simulink model "a8_real_control_smc"  (R2023b)
settings: Solver=FixedStepAuto  StartTime=0.0  StopTime=inf  RelTol=1e-3
undefined symbols (not defined in the file): dev, Main, pid_y_i, pwm_output0
libraries: simulink x15, slpidlib x6, px4Sensorslib x5, px4lib x1, px4uORBlib x1
(part 1 of 2)
settings Model: SimulationMode=external  ExtModeTrigDuration=10  Creator=UAV2  LastModifiedBy=UAV2
settings SolverCC: AlgebraicLoopSolver=TrustRegion  PositivePriorityOrder=on  MaxZcPerStep=1
settings OptimizationCC: EnhancedBackFolding=on  PassReuseOutputArgsAs=Individual arguments  ZeroExternalMemoryAtStartup=off  ZeroInternalMemoryAtStartup=off  MaxStackSize=64  OptimizeBlockOrder=speed  DifferentSizesBufferReuse=on  OptimizationCustomize=off  EfficientTunableParamExpr=on
settings DebuggingCC: ParameterTunabilityLossMsg=error  UnconnectedInputMsg=warning  UnconnectedOutputMsg=warning  UnconnectedLineMsg=warning  SymbolicDimsDataTypeCodeGenerationDiagnostic=none
settings HardwareCC: ProdBitPerPointer=32  ProdBitPerSizeT=32  ProdBitPerPtrDiffT=32  ProdLargestAtomicInteger=Long  ProdLargestAtomicFloat=Double  ProdWordSize=32  ProdLongLongMode=on  ProdHWDeviceType=ARM Compatible->ARM Cortex
settings ModelReferenceCC: EnableRefExpFcnMdlSchedulingChecks=on
settings SFSimCC: SimGenImportedTypeDefs=on  MATLABDynamicMemAlloc=off  SimTargetLang=C++
settings RTWCC: Description=Embedded Coder  SystemTargetFile=ert.tlc  HardwareBoard=PX4 Pixhawk 4  TemplateMakefile=ert_default_tmf  Toolchain=GNU Tools for PX4 Autopilots  IncludeHyperlinkInReport=on  TargetLang=C++  DLArmComputeVersion=19.05
settings CodeAppCC: ForceParamTrailComments=on  IgnoreCustomStorageClasses=off  OperatorAnnotations=on  SimulinkDataObjDesc=on  SFDataObjDesc=on  InsertBlockDesc=on
settings ERTTargetCC: ExtMode=on  ExtModeTransport=3  ExtModeStaticAlloc=on  ExtModeStaticAllocSize=1024  ExtModeMexFile=ext_xcp  ExtModeMexArgs=1 COM3 3000000  ExtModeIntrfLevel=Level2 - Open

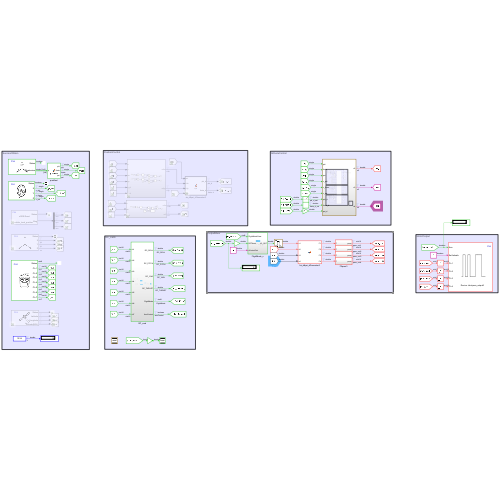
[thumbnail: Simulink's stored preview of the top-level diagram]
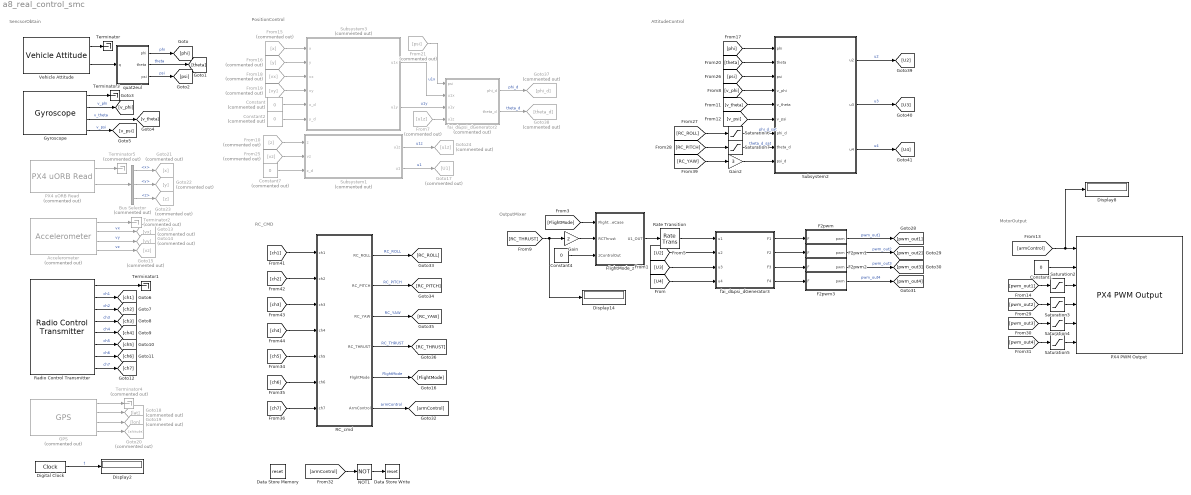
== system a8_real_control_smc ==
  note: RC_CMD
  note: PositionControl
  note: MotorOutput
  note: SencsorObtain
  note: AttitudeControl
  note: OutputMixer
  Accelerometer : px4Sensorslib/Accelerometer  Commented=on  uorbTimeStamp=off  BlockingMode=off  BlockTimeout=1e-3  sampleTime=1/250
  Bus Selector : BusSelector  Commented=on  OutputSignals=x,y,z
  Constant : Constant  Commented=on  Value=0
  Constant1 : Constant  Value=0  OutDataTypeStr=boolean
  Constant2 : Constant  Commented=on  Value=0
  Constant4 : Constant  Value=0  OutDataTypeStr=double
  Constant7 : Constant  Commented=on  Value=0
  Data Store Memory : DataStoreMemory  DataStoreName=reset  WriteAfterWriteMsg=warning  ShowAdditionalParam=off  OutDataTypeStr=boolean
  Data Store Write : DataStoreWrite  DataStoreName=reset  IndexOptions=Index vector (dialog)  Indices=1  OutputSizes=1
  Digital Clock : DigitalClock  SampleTime=0.001
  Display14 : Display
  Display2 : Display
  Display8 : Display
  F2pwm : Subsystem
  F2pwm1 : Subsystem
  F2pwm2 : Subsystem
  F2pwm3 : Subsystem
  FlightMode_z : Subsystem
  From10 : From  Commented=on  GotoTag=z
  From15 : From  Commented=on  GotoTag=x
  From16 : From  Commented=on  GotoTag=y
  From18 : From  Commented=on  GotoTag=vx
  From19 : From  Commented=on  GotoTag=vy
  From21 : From  Commented=on  GotoTag=psi
  From25 : From  Commented=on  GotoTag=vz
  From7 : From  Commented=on  GotoTag=u1z
  GPS : px4Sensorslib/GPS  Commented=on  lat=on  lon=on  alt=on  velocity=off  course=off  gpsfix=off  numsat=off  timestamp_utc=off  BlockingMode=off  BlockTimeout=1e-3  dop=off  vel_ned=off  alt_ellipsoid=off  jamm_ind=off  timestamp=off  sampleTime=1/250
  Gain : Gain  Gain=2
  Gain2 : Gain  Gain=3
  Goto13 : Goto  Commented=on  GotoTag=vx
  Goto14 : Goto  Commented=on  GotoTag=vy
  Goto15 : Goto  Commented=on  GotoTag=vz
  Goto17 : Goto  Commented=on  GotoTag=U1
  Goto18 : Goto  Commented=on  GotoTag=lat
  Goto19 : Goto  Commented=on  GotoTag=lon
  Goto20 : Goto  Commented=on  GotoTag=altitude
  Goto21 : Goto  Commented=on  GotoTag=x
  Goto22 : Goto  Commented=on  GotoTag=y
  Goto23 : Goto  Commented=on  GotoTag=z
  Goto24 : Goto  Commented=on  GotoTag=u1z
  Goto37 : Goto  Commented=on  GotoTag=phi_d
  Goto38 : Goto  Commented=on  GotoTag=theta_d
  Gyroscope : px4Sensorslib/Gyroscope  uorbTimeStamp=off  BlockingMode=off  BlockTimeout=1e-3  sampleTime=1/250
  NOT1 : Logic  Operator=NOT  IconShape=distinctive  AllPortsSameDT=off  OutDataTypeStr=boolean
  PX4 PWM Output : px4lib/PX4 PWM Output  pwmDevice=Main (/dev/pwm_output0)  pwmChannel1_=on  pwmChannel2_=on  pwmChannel3_=on  pwmChannel4_=on  pwmChannel5_=off  pwmChannel6_=off  pwmChannel7_=off  pwmChannel8_=off  forceTerminateFailsafe=off  outputErrorStatus=off
  PX4 uORB Read : px4uORBlib/PX4 uORB Read  Commented=on  uORBTopic=vehicle_local_position  selectInstance=actuator_armed  SampleTime=1/250  BlockingMode=off  BlockTimeout=1e-3
  RC_cmd : Subsystem  Tag=attitudeControl
  Radio Control Transmitter : px4Sensorslib/Radio Control Transmitter  channel1=on  channel2=on  channel3=on  channel4=on  channel5=on  channel6=on  channel7=on  channel8=off  channel_count=off  rssi=off  rc_input_source=off  timestamp_last_signal=off  time_stamp=off  sampleTime=1/250  BlockingMode=off  BlockTimeout=5
  Rate Transition : RateTransition
  Saturation{2..5} (4 alike) : Saturate  UpperLimit=2000  LowerLimit=1050
  Saturation6 : Saturate
  Saturation7 : Saturate
  Subsystem1 : Subsystem  Commented=on
  Subsystem2 : Subsystem
  Subsystem3 : Subsystem  Commented=on
  Terminator : Terminator
  Terminator1 : Terminator
  Terminator2 : Terminator  Commented=on
  Terminator3 : Terminator
  Terminator4 : Terminator  Commented=on
  Terminator5 : Terminator  Commented=on
  Vehicle Attitude : px4Sensorslib/Vehicle Attitude  rollRate=off  pitchRate=off  yawRate=off  quaternion=on  uorbTimeStamp=off  BlockingMode=off  BlockTimeout=0.001  sampleTime=1/250
  fai_d&psi_dGenerator2 : MATLAB Function  Commented=on  TreatAsAtomicUnit=on
  fai_d&psi_dGenerator3 : MATLAB Function  TreatAsAtomicUnit=on
  quat2eul : MATLAB Function  TreatAsAtomicUnit=on
  wires:
  Accelerometer/3 -> Goto14/1  "vy"
  [armControl] -> NOT1/1
  From19/1 -> Subsystem3/4(vy)
  Constant1/1 -> PX4 PWM Output/2
  [ch3] -> RC_cmd/3(ch3)
  Gyroscope/3 -> [v_theta]  "v_theta"
  [ch2] -> RC_cmd/2(ch2)
  quat2eul/2(theta) -> [theta]  "theta"
  [pwm_out3] -> Saturation4/1
  Constant2/1 -> Subsystem3/6(y_d)
  Gain/1 -> FlightMode_z/2(RCThrust)
  Constant/1 -> Subsystem3/5(x_d)
  fai_d&psi_dGenerator3/3(F3) -> F2pwm2/1(F)
  [ch6] -> RC_cmd/6(ch6)
  Bus Selector/3 -> Goto23/1  "<z>"
  [ch4] -> RC_cmd/4(ch4)
  FlightMode_z/1(U1_OUT) -> Rate Transition/1
  RC_cmd/5(FlightMode) -> [FlightMode]  "FlightMode"
  fai_d&psi_dGenerator2/2(theta_d) -> Goto38/1  "theta_d"
  Accelerometer/1 -> Terminator2/1
  Constant4/1 -> FlightMode_z/3(zControlOut)
  RC_cmd/6(ArmControl) -> [armControl]  "armControl"
  From16/1 -> Subsystem3/2(y)
  RC_cmd/1(RC_ROLL) -> [RC_ROLL]  "RC_ROLL"
  [RC_THRUST] -> Display14/1, Gain/1
  quat2eul/1(phi) -> [phi]  "phi"
  NOT1/1 -> Data Store Write/1
  RC_cmd/4(RC_THRUST) -> [RC_THRUST]  "RC_THRUST"
  Vehicle Attitude/2 -> quat2eul/1(q)
  RC_cmd/2(RC_PITCH) -> [RC_PITCH]  "RC_PITCH"
  RC_cmd/3(RC_YAW) -> [RC_YAW]  "RC_YAW"
  [ch5] -> RC_cmd/5(ch5)
  F2pwm/1(pwm) -> [pwm_out1]  "pwm_out1"
  [ch7] -> RC_cmd/7(ch7)
  [pwm_out1] -> Saturation2/1
  fai_d&psi_dGenerator3/2(F2) -> F2pwm1/1(F)
  [ch1] -> RC_cmd/1(ch1)
  F2pwm1/1(pwm) -> [pwm_out2]  "pwm_out2"
  [pwm_out2] -> Saturation3/1
  Radio Control Transmitter/2 -> [ch1]  "ch1"
  fai_d&psi_dGenerator3/4(F4) -> F2pwm3/1(F)
  Accelerometer/2 -> Goto13/1  "vx"
  fai_d&psi_dGenerator3/1(F1) -> F2pwm/1(F)
  [pwm_out4] -> Saturation5/1
  Accelerometer/4 -> Goto15/1  "vz"
  Subsystem3/1(u1x) -> fai_d&psi_dGenerator2/2(u1x)  "u1x"
  Subsystem3/2(u1y) -> fai_d&psi_dGenerator2/3(u1y)  "u1y"
  From18/1 -> Subsystem3/3(vx)
  From21/1 -> fai_d&psi_dGenerator2/1(psi)
  Bus Selector/2 -> Goto22/1  "<y>"
  Radio Control Transmitter/5 -> [ch4]  "ch4"
  Radio Control Transmitter/6 -> [ch5]  "ch5"
  Radio Control Transmitter/8 -> [ch7]  "ch7"
  Gyroscope/1 -> Terminator3/1
  Radio Control Transmitter/3 -> [ch2]  "ch2"
  PX4 uORB Read/2 -> Bus Selector/1
  Radio Control Transmitter/7 -> [ch6]  "ch6"
  GPS/4 -> Goto20/1
  Bus Selector/1 -> Goto21/1  "<x>"
  GPS/1 -> Terminator4/1
  From15/1 -> Subsystem3/1(x)
  quat2eul/3(psi) -> [psi]  "psi"
  Vehicle Attitude/1 -> Terminator/1
  Gyroscope/4 -> [v_psi]  "v_psi"
  F2pwm3/1(pwm) -> [pwm_out4]  "pwm_out4"
  [armControl] -> Display8/1, PX4 PWM Output/1
  Radio Control Transmitter/4 -> [ch3]  "ch3"
  fai_d&psi_dGenerator2/1(phi_d) -> Goto37/1  "phi_d"
  Digital Clock/1 -> Display2/1  "t"
  GPS/2 -> Goto18/1
  Radio Control Transmitter/1 -> Terminator1/1
  PX4 uORB Read/1 -> Terminator5/1
  Gyroscope/2 -> [v_phi]  "v_phi"
  GPS/3 -> Goto19/1
  F2pwm2/1(pwm) -> [pwm_out3]  "pwm_out3"
  [FlightMode] -> FlightMode_z/1(FlightModeCase)
  Saturation2/1 -> PX4 PWM Output/3
  Saturation3/1 -> PX4 PWM Output/4
  Saturation4/1 -> PX4 PWM Output/5
  Saturation5/1 -> PX4 PWM Output/6
  Rate Transition/1 -> fai_d&psi_dGenerator3/1(u1)
  [U2] -> fai_d&psi_dGenerator3/2(u2)
  Subsystem1/2(u1) -> Goto17/1  "u1"
  From10/1 -> Subsystem1/1(z)
  From25/1 -> Subsystem1/2(vz)
  Constant7/1 -> Subsystem1/3(z_d)
  Subsystem1/1(u1z) -> Goto24/1  "u1z"
  From7/1 -> fai_d&psi_dGenerator2/4(u1z)
  [RC_PITCH] -> Saturation7/1
  [RC_ROLL] -> Saturation6/1
  [RC_YAW] -> Gain2/1
  Gain2/1 -> Subsystem2/9(psi_d)
  Saturation6/1 -> Subsystem2/7(phi_d)  "phi_d_sat"
  Saturation7/1 -> Subsystem2/8(theta_d)  "theta_d_sat"
  [phi] -> Subsystem2/1(phi)
  [theta] -> Subsystem2/2(theta)
  [psi] -> Subsystem2/3(psi)
  [v_phi] -> Subsystem2/4(v_phi)
  [v_theta] -> Subsystem2/5(v_theta)
  [v_psi] -> Subsystem2/6(v_psi)
  Subsystem2/1(u2) -> [U2]  "u2"
  Subsystem2/2(u3) -> [U3]  "u3"
  Subsystem2/3(u4) -> [U4]  "u4"
  [U3] -> fai_d&psi_dGenerator3/3(u3)
  [U4] -> fai_d&psi_dGenerator3/4(u4)

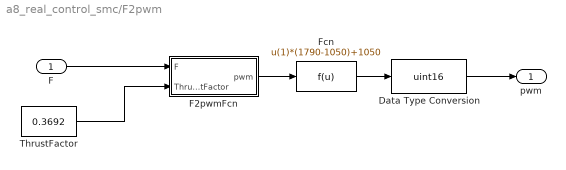
== system a8_real_control_smc/F2pwm ==
  F : Inport
  Data Type Conversion : DataTypeConversion  OutDataTypeStr=uint16  SaturateOnIntegerOverflow=off  RndMeth=Floor
  F2pwmFcn : Subsystem
  Fcn : Fcn  Expr=u(1)*(1790-1050)+1050
  ThrustFactor : Constant  Value=0.3692
  pwm : Outport  OutDataTypeStr=uint16  VectorParamsAs1DForOutWhenUnconnected=off
  wires:
  F/1 -> F2pwmFcn/1(F)
  ThrustFactor/1 -> F2pwmFcn/2(ThrustFactor)
  F2pwmFcn/1(pwm) -> Fcn/1
  Fcn/1 -> Data Type Conversion/1
  Data Type Conversion/1 -> pwm/1

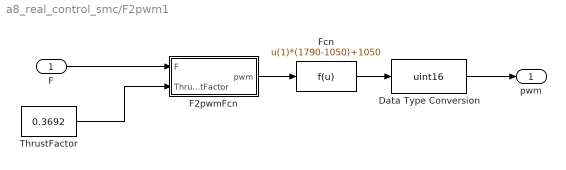
== system a8_real_control_smc/F2pwm1 ==
  F : Inport
  Data Type Conversion : DataTypeConversion  OutDataTypeStr=uint16  SaturateOnIntegerOverflow=off  RndMeth=Floor
  F2pwmFcn : Subsystem
  Fcn : Fcn  Expr=u(1)*(1790-1050)+1050
  ThrustFactor : Constant  Value=0.3692
  pwm : Outport  OutDataTypeStr=uint16  VectorParamsAs1DForOutWhenUnconnected=off
  wires:
  Data Type Conversion/1 -> pwm/1
  Fcn/1 -> Data Type Conversion/1
  F2pwmFcn/1(pwm) -> Fcn/1
  ThrustFactor/1 -> F2pwmFcn/2(ThrustFactor)
  F/1 -> F2pwmFcn/1(F)

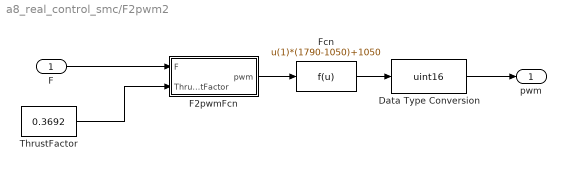
== system a8_real_control_smc/F2pwm2 ==
  F : Inport
  Data Type Conversion : DataTypeConversion  OutDataTypeStr=uint16  SaturateOnIntegerOverflow=off  RndMeth=Floor
  F2pwmFcn : Subsystem
  Fcn : Fcn  Expr=u(1)*(1790-1050)+1050
  ThrustFactor : Constant  Value=0.3692
  pwm : Outport  OutDataTypeStr=uint16  VectorParamsAs1DForOutWhenUnconnected=off
  wires:
  F/1 -> F2pwmFcn/1(F)
  ThrustFactor/1 -> F2pwmFcn/2(ThrustFactor)
  F2pwmFcn/1(pwm) -> Fcn/1
  Fcn/1 -> Data Type Conversion/1
  Data Type Conversion/1 -> pwm/1

== system a8_real_control_smc/F2pwm3 ==
  F : Inport
  Data Type Conversion : DataTypeConversion  OutDataTypeStr=uint16  SaturateOnIntegerOverflow=off  RndMeth=Floor
  F2pwmFcn : Subsystem
  Fcn : Fcn  Expr=u(1)*(1790-1050)+1050
  ThrustFactor : Constant  Value=0.3692
  pwm : Outport  OutDataTypeStr=uint16  VectorParamsAs1DForOutWhenUnconnected=off
  wires:
  Data Type Conversion/1 -> pwm/1
  Fcn/1 -> Data Type Conversion/1
  F2pwmFcn/1(pwm) -> Fcn/1
  ThrustFactor/1 -> F2pwmFcn/2(ThrustFactor)
  F/1 -> F2pwmFcn/1(F)

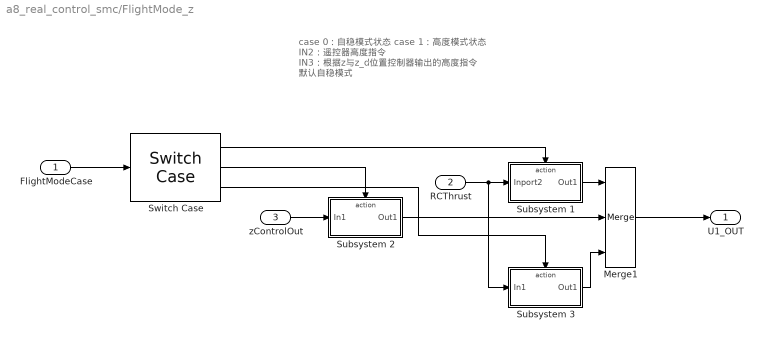
== system a8_real_control_smc/FlightMode_z ==
  note: case 0：自稳模式状态
      | case 1：高度模式状态
      | IN2：遥控器高度指令
      | IN3：根据z与z_d位置控制器输出的高度指令
      | 默认自稳模式
  FlightModeCase : Inport
  RCThrust : Inport  Port=2
  zControlOut : Inport  Port=3
  Merge1 : Merge  Inputs=3
  Subsystem 1 : Subsystem  TreatAsAtomicUnit=on
  Subsystem 2 : Subsystem  TreatAsAtomicUnit=on
  Subsystem 3 : Subsystem  TreatAsAtomicUnit=on
  Switch Case : SwitchCase  CaseConditions={0,1}
  U1_OUT : Outport  VectorParamsAs1DForOutWhenUnconnected=off
  wires:
  Switch Case/2 -> Subsystem 2/Action
  Subsystem 2/1(Out1) -> Merge1/2
  RCThrust/1 -> Subsystem 1/1(Inport2), Subsystem 3/1(In1)
  Switch Case/3 -> Subsystem 3/Action
  Subsystem 1/1(Out1) -> Merge1/1
  Switch Case/1 -> Subsystem 1/Action
  Subsystem 3/1(Out1) -> Merge1/3
  zControlOut/1 -> Subsystem 2/1(In1)
  FlightModeCase/1 -> Switch Case/1
  Merge1/1 -> U1_OUT/1

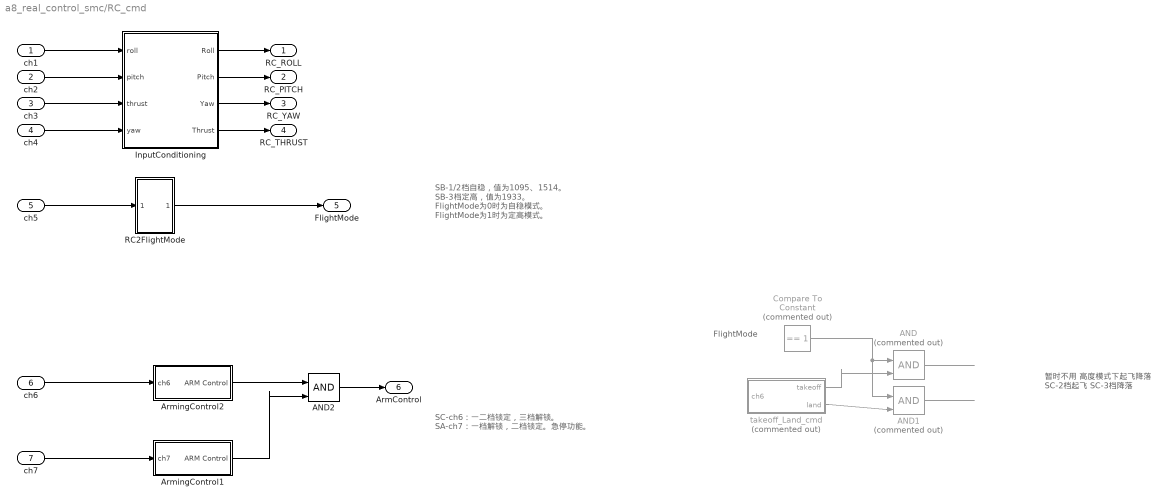
== system a8_real_control_smc/RC_cmd ==
  note: 暂时不用
      | 高度模式下起飞降落
      | SC-2档起飞
      | SC-3档降落
  note: SB-1/2档自稳，值为1095、1514。
      | SB-3档定高，值为1933。
      | FlightMode为0时为自稳模式。
      | FlightMode为1时为定高模式。
  note: FlightMode
  note: SC-ch6：一二档锁定，三档解锁。
      | SA-ch7：一档解锁，二档锁定。急停功能。
  ch1 : Inport  OutDataTypeStr=uint16
  ch2 : Inport  Port=2  OutDataTypeStr=uint16
  ch3 : Inport  Port=3  OutDataTypeStr=uint16
  ch4 : Inport  Port=4  OutDataTypeStr=uint16
  ch5 : Inport  Port=5  OutDataTypeStr=uint16
  ch6 : Inport  Port=6  OutDataTypeStr=uint16
  ch7 : Inport  Port=7  OutDataTypeStr=uint16
  AND : Logic  Commented=on  IconShape=distinctive  AllPortsSameDT=off  OutDataTypeStr=boolean
  AND1 : Logic  Commented=on  IconShape=distinctive  AllPortsSameDT=off  OutDataTypeStr=boolean
  AND2 : Logic  IconShape=distinctive  AllPortsSameDT=off  OutDataTypeStr=boolean
  ArmingControl1 : Subsystem
  ArmingControl2 : Subsystem
  Compare To Constant : simulink/Logic and Bit Operations/Compare To Constant  Commented=on  relop===  const=1  OutDataTypeStr=boolean
  InputConditioning : Subsystem
  RC2FlightMode : Subsystem
  takeoff_Land_cmd : Subsystem  Commented=on
  RC_ROLL : Outport
  RC_PITCH : Outport  Port=2
  RC_YAW : Outport  Port=3
  RC_THRUST : Outport  Port=4
  FlightMode : Outport  Port=5
  ArmControl : Outport  Port=6
  wires:
  ch7/1 -> ArmingControl1/1(ch7)
  ch4/1 -> InputConditioning/4(yaw)
  ch1/1 -> InputConditioning/1(roll)
  ch2/1 -> InputConditioning/2(pitch)
  ch3/1 -> InputConditioning/3(thrust)
  InputConditioning/1(Roll) -> RC_ROLL/1
  InputConditioning/2(Pitch) -> RC_PITCH/1
  InputConditioning/3(Yaw) -> RC_YAW/1
  InputConditioning/4(Thrust) -> RC_THRUST/1
  takeoff_Land_cmd/1(takeoff) -> AND/2
  AND/1 -> ?
  AND1/1 -> ?
  takeoff_Land_cmd/2(land) -> AND1/2
  ch5/1 -> RC2FlightMode/1(In1)
  RC2FlightMode/1(Out1) -> FlightMode/1
  Compare To Constant/1 -> AND1/1, AND/1
  ch6/1 -> ArmingControl2/1(ch6)
  ArmingControl2/1(ARM Control) -> AND2/1
  ArmingControl1/1(ARM Control) -> AND2/2
  AND2/1 -> ArmControl/1

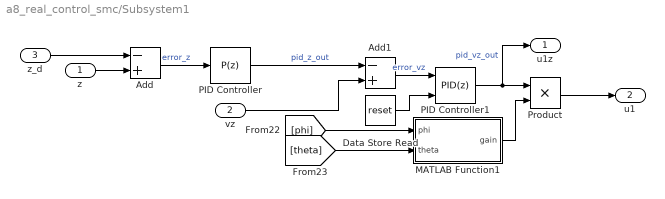
== system a8_real_control_smc/Subsystem1 ==
  z : Inport
  vz : Inport  Port=2
  z_d : Inport  Port=3
  Add : Sum  Inputs=-+
  Add1 : Sum  Inputs=-+
  Data Store Read : DataStoreRead  DataStoreName=reset  IndexOptions=Index vector (dialog)  Indices=1  OutputSizes=1
  MATLAB Function1 : MATLAB Function  TreatAsAtomicUnit=on
  PID Controller : slpidlib/PID Controller  Controller=P  Form=Parallel  TimeDomain=Discrete-time  UseExternalTs=off  SampleTime=-1  IntegratorMethod=Forward Euler  FilterMethod=Forward Euler  ControllerParametersSource=internal  P=1.5  I=1.33332542389365  UseKiTs=off  D=0.947452162670561  N=36.1071689779307  UseFilter=on  TunerSelectOption=Transfer Function Based (PID Tuner App)  InitialConditionSource=internal  InitialConditionForIntegrator=0  InitialConditionForFilter=0  DifferentiatorICPrevScaledInput=0  ExternalReset=none  TrackingMode=off  Kt=1  LimitOutput=on  SatLimitsSource=internal  UpperSaturationLimit=10  LowerSaturationLimit=-10  LinearizeAsGain=off  AntiWindupMode=none  Kb=1  LimitIntegrator=off  UpperIntegratorSaturationLimit=inf  LowerIntegratorSaturationLimit=-inf  POutMin=[]  POutMax=[]  IOutMin=[]  IOutMax=[]  DOutMin=[]  DOutMax=[]  NOutMin=[]  NOutMax=[]  SumOutMin=[]  SumOutMax=[]  SaturationOutMin=[]  SaturationOutMax=[]  PParamMin=[]  PParamMax=[]  IParamMin=[]  IParamMax=[]  DParamMin=[]  DParamMax=[]  NParamMin=[]  NParamMax=[]  KbParamMin=[]  KbParamMax=[]  KtParamMin=[]  KtParamMax=[]  KbOutMin=[]  KbOutMax=[]  KtOutMin=[]  KtOutMax=[]  IntegratorOutMin=[]  IntegratorOutMax=[]  FilterOutMin=[]  FilterOutMax=[]  SumI1OutMin=[]  SumI1OutMax=[]  SumI2OutMin=[]  SumI2OutMax=[]  SumI3OutMin=[]  SumI3OutMax=[]  SumI4OutMin=[]  SumI4OutMax=[]  SumDOutMin=[]  SumDOutMax=[]  DifferentiatorOutMin=[]  DifferentiatorOutMax=[]  FilterDiffOutCoefMin=[]  FilterDiffOutCoefMax=[]  ReciprocalOutMin=[]  ReciprocalOutMax=[]  SumDenOutMin=[]  SumDenOutMax=[]  SumNumOutMin=[]  SumNumOutMax=[]  DivideOutMin=[]  DivideOutMax=[]  UdiffTsProdOutMin=[]  UdiffTsProdOutMax=[]  NTsProdOutMin=[]  NTsProdOutMax=[]  UintegralTsProdOutMin=[]  UintegralTsProdOutMax=[]  UngainTsProdOutMin=[]  UngainTsProdOutMax=[]  ClampingZeroOutDataTypeStr=Inherit: Inherit via back propagation  ClampingZeroOutMin=[]  ClampingZeroOutMax=[]  FilterDenConstantOutDataTypeStr=Inherit: Inherit via back propagation  FilterDenConstantOutMin=[]  FilterDenConstantOutMax=[]  PCopyOutDataTypeStr=Inherit: Inherit via back propagation  PCopyOutMin=[]  PCopyOutMax=[]  NCopyOutDataTypeStr=Inherit: Inherit via back propagation  NCopyOutMin=[]  NCopyOutMax=[]  IntegratorContinuousStateAttributes=''  IntegratorStateMustResolveToSignalObject=off  IntegratorRTWStateStorageClass=Auto  FilterContinuousStateAttributes=''  FilterStateMustResolveToSignalObject=off  FilterRTWStateStorageClass=Auto  ParallelPVariant=InternalParameters  IdealPVariant=Disabled  IVariant=Disabled  DVariant=Disabled  IntegratorVariant=Disabled  SatVariant=Enabled  AWVariant=Disabled  PCopyVariant=Disabled  TRVariant=Disabled  FdbkBlocksVariant=Forward  IdealPFdbkVariant=Disabled  SatFdbkVariant=Disabled  DerivativeFilterVariant=Disabled  NVariant=Disabled  NCopyVariant=Disabled_SignalSpec  FilterICVariant=Disabled  IntegratorICVariant=Disabled  ExternalResetVariant=Disabled  TRSumVariant=Passthrough  SumFdbkVariant=Disabled  SumVariant=Passthrough_P  TsampFilterVariant=InternalTs  TsampNgainVariant=Passthrough  TsampIntegralVariant=Disabled_SignalSpec  ExternalSaturationOutDataTypeStr=Inherit: Same as second input
  PID Controller1 : slpidlib/PID Controller  Controller=PID  Form=Parallel  TimeDomain=Discrete-time  UseExternalTs=off  SampleTime=-1  IntegratorMethod=Forward Euler  FilterMethod=Forward Euler  ControllerParametersSource=internal  P=0.6  I=0.3  UseKiTs=off  D=0  N=10  UseFilter=on  TunerSelectOption=Transfer Function Based (PID Tuner App)  InitialConditionSource=internal  InitialConditionForIntegrator=0  InitialConditionForFilter=0  DifferentiatorICPrevScaledInput=0  ExternalReset=level  TrackingMode=off  Kt=1  LimitOutput=on  SatLimitsSource=internal  UpperSaturationLimit=1  LowerSaturationLimit=0  LinearizeAsGain=off  AntiWindupMode=none  Kb=1  LimitIntegrator=off  UpperIntegratorSaturationLimit=0.1  LowerIntegratorSaturationLimit=-0.1  POutMin=[]  POutMax=[]  IOutMin=[]  IOutMax=[]  DOutMin=[]  DOutMax=[]  NOutMin=[]  NOutMax=[]  SumOutMin=[]  SumOutMax=[]  SaturationOutMin=[]  SaturationOutMax=[]  PParamMin=[]  PParamMax=[]  IParamMin=[]  IParamMax=[]  DParamMin=[]  DParamMax=[]  NParamMin=[]  NParamMax=[]  KbParamMin=[]  KbParamMax=[]  KtParamMin=[]  KtParamMax=[]  KbOutMin=[]  KbOutMax=[]  KtOutMin=[]  KtOutMax=[]  IntegratorOutMin=[]  IntegratorOutMax=[]  FilterOutMin=[]  FilterOutMax=[]  SumI1OutMin=[]  SumI1OutMax=[]  SumI2OutMin=[]  SumI2OutMax=[]  SumI3OutMin=[]  SumI3OutMax=[]  SumI4OutMin=[]  SumI4OutMax=[]  SumDOutMin=[]  SumDOutMax=[]  DifferentiatorOutMin=[]  DifferentiatorOutMax=[]  FilterDiffOutCoefMin=[]  FilterDiffOutCoefMax=[]  ReciprocalOutMin=[]  ReciprocalOutMax=[]  SumDenOutMin=[]  SumDenOutMax=[]  SumNumOutMin=[]  SumNumOutMax=[]  DivideOutMin=[]  DivideOutMax=[]  UdiffTsProdOutMin=[]  UdiffTsProdOutMax=[]  NTsProdOutMin=[]  NTsProdOutMax=[]  UintegralTsProdOutMin=[]  UintegralTsProdOutMax=[]  UngainTsProdOutMin=[]  UngainTsProdOutMax=[]  ClampingZeroOutDataTypeStr=Inherit: Inherit via back propagation  ClampingZeroOutMin=[]  ClampingZeroOutMax=[]  FilterDenConstantOutDataTypeStr=Inherit: Inherit via back propagation  FilterDenConstantOutMin=[]  FilterDenConstantOutMax=[]  PCopyOutDataTypeStr=Inherit: Inherit via back propagation  PCopyOutMin=[]  PCopyOutMax=[]  NCopyOutDataTypeStr=Inherit: Inherit via back propagation  NCopyOutMin=[]  NCopyOutMax=[]  IntegratorContinuousStateAttributes=''  IntegratorStateMustResolveToSignalObject=off  IntegratorRTWStateStorageClass=Auto  FilterContinuousStateAttributes=''  FilterStateMustResolveToSignalObject=off  FilterRTWStateStorageClass=Auto  ParallelPVariant=InternalParameters  IdealPVariant=Disabled  IVariant=InternalParameters  DVariant=InternalParameters  IntegratorVariant=Discrete  SatVariant=Enabled  AWVariant=Passthrough  PCopyVariant=Disabled  TRVariant=Disabled  FdbkBlocksVariant=Forward  IdealPFdbkVariant=Disabled  SatFdbkVariant=Disabled  DerivativeFilterVariant=ForwardEulerFilter  NVariant=InternalParameters  NCopyVariant=Disabled  FilterICVariant=InternalICsFilter  IntegratorICVariant=InternalICs  ExternalResetVariant=ExternalReset  TRSumVariant=Passthrough  SumFdbkVariant=Disabled  SumVariant=Sum_PID  TsampFilterVariant=InternalTs  TsampNgainVariant=Passthrough  TsampIntegralVariant=Disabled_SignalSpec  ExternalSaturationOutDataTypeStr=Inherit: Same as second input
  Product : Product
  u1z : Outport
  u1 : Outport  Port=2
  wires:
  z/1 -> Add/2
  z_d/1 -> Add/1
  Data Store Read/1 -> PID Controller1/2
  Add1/1 -> PID Controller1/1  "error_vz"
  PID Controller/1 -> Add1/1  "pid_z_out"
  PID Controller1/1 -> Product/1, u1z/1  "pid_vz_out"
  vz/1 -> Add1/2
  MATLAB Function1/1(gain) -> Product/2
  [theta] -> MATLAB Function1/2(theta)
  Product/1 -> u1/1
  Add/1 -> PID Controller/1  "error_z"
  [phi] -> MATLAB Function1/1(phi)

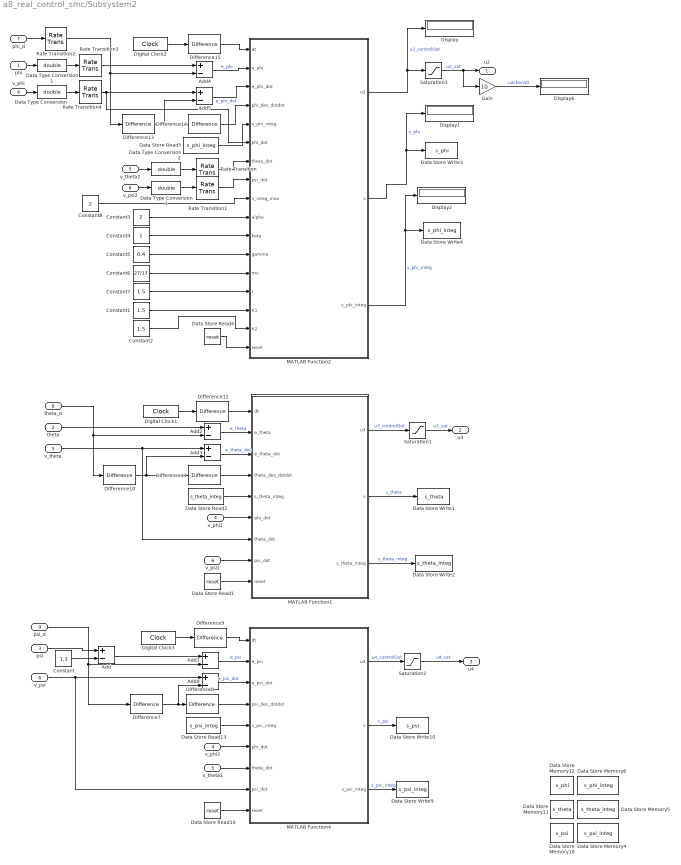
== system a8_real_control_smc/Subsystem2 ==
  phi : Inport
  theta : Inport  Port=2
  psi : Inport  Port=3
  v_phi : Inport  Port=4
  v_theta : Inport  Port=5
  v_psi : Inport  Port=6
  phi_d : Inport  Port=7
  theta_d : Inport  Port=8
  psi_d : Inport  Port=9
  Add{,1..5,9} (7 alike) : Sum  Inputs=+-
  Constant : Constant  Value=1.1
  Constant1 : Constant  Value=1.5
  Constant2 : Constant  Value=1.5
  Constant3 : Constant  Value=2
  Constant4 : Constant
  Constant5 : Constant  Value=0.4
  Constant6 : Constant  Value=27/17
  Constant7 : Constant  Value=1.5
  Constant8 : Constant  Value=2
  Data Store Memory10 : DataStoreMemory  DataStoreName=s_psi  WriteAfterWriteMsg=warning  ShowAdditionalParam=off  OutDataTypeStr=double
  Data Store Memory11 : DataStoreMemory  DataStoreName=s_theta  WriteAfterWriteMsg=warning  ShowAdditionalParam=off  OutDataTypeStr=double
  Data Store Memory12 : DataStoreMemory  DataStoreName=s_phi  WriteAfterWriteMsg=warning  ShowAdditionalParam=off  OutDataTypeStr=double
  Data Store Memory4 : DataStoreMemory  DataStoreName=s_psi_integ  WriteAfterWriteMsg=warning  ShowAdditionalParam=off  OutDataTypeStr=double
  Data Store Memory5 : DataStoreMemory  DataStoreName=s_theta_integ  WriteAfterWriteMsg=warning  ShowAdditionalParam=off  OutDataTypeStr=double
  Data Store Memory6 : DataStoreMemory  DataStoreName=s_phi_integ  WriteAfterWriteMsg=warning  ShowAdditionalParam=off  OutDataTypeStr=double
  Data Store Read1 : DataStoreRead  DataStoreName=reset  IndexOptions=Index vector (dialog)  Indices=1  OutputSizes=1
  Data Store Read10 : DataStoreRead  DataStoreName=reset  IndexOptions=Index vector (dialog)  Indices=1  OutputSizes=1
  Data Store Read13 : DataStoreRead  DataStoreName=s_psi_integ  IndexOptions=Index vector (dialog)  Indices=1  OutputSizes=1
  Data Store Read2 : DataStoreRead  DataStoreName=s_theta_integ  IndexOptions=Index vector (dialog)  Indices=1  OutputSizes=1
  Data Store Read4 : DataStoreRead  DataStoreName=reset  IndexOptions=Index vector (dialog)  Indices=1  OutputSizes=1
  Data Store Read5 : DataStoreRead  DataStoreName=s_phi_integ  IndexOptions=Index vector (dialog)  Indices=1  OutputSizes=1
  Data Store Write1 : DataStoreWrite  DataStoreName=s_theta  IndexOptions=Index vector (dialog)  Indices=1  OutputSizes=1
  Data Store Write10 : DataStoreWrite  DataStoreName=s_psi  IndexOptions=Index vector (dialog)  Indices=1  OutputSizes=1
  Data Store Write2 : DataStoreWrite  DataStoreName=s_theta_integ  IndexOptions=Index vector (dialog)  Indices=1  OutputSizes=1
  Data Store Write3 : DataStoreWrite  DataStoreName=s_phi  IndexOptions=Index vector (dialog)  Indices=1  OutputSizes=1
  Data Store Write4 : DataStoreWrite  DataStoreName=s_phi_integ  IndexOptions=Index vector (dialog)  Indices=1  OutputSizes=1
  Data Store Write9 : DataStoreWrite  DataStoreName=s_psi_integ  IndexOptions=Index vector (dialog)  Indices=1  OutputSizes=1
  Data Type Conversion{,1..3} (4 alike) : DataTypeConversion  OutDataTypeStr=double  SaturateOnIntegerOverflow=off  RndMeth=Floor
  Difference{7..15} (9 alike) : simulink/Discrete/Difference  ICPrevInput=0.0  OutMin=[]  OutMax=[]  OutDataType=fixdt(1, 16)  OutScaling=2^-10  DoSatur=off
  Digital Clock1 : DigitalClock  SampleTime=0.001
  Digital Clock2 : DigitalClock  SampleTime=0.001
  Digital Clock3 : DigitalClock  SampleTime=0.001
  Display{,1..2,6} (4 alike) : Display
  Gain : Gain  Gain=10
  MATLAB Function1 : MATLAB Function  TreatAsAtomicUnit=on
  MATLAB Function2 : MATLAB Function  TreatAsAtomicUnit=on
  MATLAB Function4 : MATLAB Function  TreatAsAtomicUnit=on
  Rate Transition{,1..4} (5 alike) : RateTransition
  Saturation1 : Saturate  UpperLimit=0.1  LowerLimit=-0.1
  Saturation2 : Saturate  UpperLimit=0.2  LowerLimit=-0.2
  Saturation3 : Saturate  UpperLimit=0.2  LowerLimit=-0.2
  v_phi1 : InportShadow  Port=4
  v_phi2 : InportShadow  Port=4
  v_psi1 : InportShadow  Port=6
  v_psi2 : InportShadow  Port=6
  v_theta1 : InportShadow  Port=5
  v_theta2 : InportShadow  Port=5
  u2 : Outport
  u3 : Outport  Port=2
  u4 : Outport  Port=3
  wires:
  Data Store Read10/1 -> MATLAB Function4/9(reset)
  Data Store Read13/1 -> MATLAB Function4/5("s_psi_integ ")
  MATLAB Function4/3(s_psi_integ) -> Data Store Write9/1  "s_psi_integ"
  Saturation2/1 -> u4/1  "u4_sat"
  Add9/1 -> MATLAB Function4/3(e_psi_dot)  "e_psi_dot"
  Difference7/1 -> Add9/2, Difference8/1
  Difference8/1 -> MATLAB Function4/4(psi_des_dotdot)
  Difference9/1 -> MATLAB Function4/1(dt)
  MATLAB Function4/2(s) -> Data Store Write10/1  "s_psi"
  MATLAB Function4/1(u4) -> Saturation2/1  "u4_controlOut"
  Digital Clock3/1 -> Difference9/1
  Add1/1 -> MATLAB Function4/2(e_psi)  "e_psi"
  Difference12/1 -> MATLAB Function1/1(dt)
  Digital Clock1/1 -> Difference12/1
  Difference11/1 -> MATLAB Function1/4(theta_des_dotdot)
  MATLAB Function1/1(u3) -> Saturation1/1  "u3_controlOut"
  Data Store Read2/1 -> MATLAB Function1/5("s_theta_integ ")
  MATLAB Function1/2(s) -> Data Store Write1/1  "s_theta"
  Difference10/1 -> Add3/2, Difference11/1
  Data Store Read1/1 -> MATLAB Function1/9(reset)
  Add2/1 -> MATLAB Function1/2(e_theta)  "e_theta"
  Add3/1 -> MATLAB Function1/3(e_theta_dot)  "e_theta_dot"
  MATLAB Function1/3(s_theta_integ) -> Data Store Write2/1  "s_theta_integ"
  theta/1 -> Add2/1
  Saturation3/1 -> Gain/1, u2/1  "u2_sat"
  phi/1 -> Data Type Conversion1/1
  Difference13/1 -> Add5/2, Difference14/1
  Data Store Read4/1 -> MATLAB Function2/17(reset)
  MATLAB Function2/1(u2) -> Display/1, Saturation3/1  "u2_controlOut"
  Data Store Read5/1 -> MATLAB Function2/5("s_phi_integ ")
  Difference14/1 -> MATLAB Function2/4(phi_des_dotdot)
  Digital Clock2/1 -> Difference15/1
  Difference15/1 -> MATLAB Function2/1(dt)
  Add5/1 -> MATLAB Function2/3(e_phi_dot)  "e_phi_dot"
  MATLAB Function2/2(s) -> Display1/1, Data Store Write3/1  "s_phi"
  Add4/1 -> MATLAB Function2/2(e_phi)  "e_phi"
  MATLAB Function2/3(s_phi_integ) -> Display2/1, Data Store Write4/1  "s_phi_integ"
  v_phi/1 -> Data Type Conversion/1
  v_theta/1 -> Add3/1, MATLAB Function1/7(theta_dot)
  v_psi/1 -> Add9/1, MATLAB Function4/8(psi_dot)
  v_phi1/1 -> MATLAB Function1/6(phi_dot)
  v_theta2/1 -> Data Type Conversion2/1
  v_psi2/1 -> Data Type Conversion3/1
  v_psi1/1 -> MATLAB Function1/8(psi_dot)
  v_phi2/1 -> MATLAB Function4/6(phi_dot)
  v_theta1/1 -> MATLAB Function4/7(theta_dot)
  Saturation1/1 -> u3/1  "u3_sat"
  psi_d/1 -> Difference7/1, Add1/2
  theta_d/1 -> Difference10/1, Add2/2
  phi_d/1 -> Rate Transition2/1
  psi/1 -> Add/1
  Constant/1 -> Add/2
  Add/1 -> Add1/1
  Rate Transition/1 -> MATLAB Function2/7(theta_dot)
  Rate Transition1/1 -> MATLAB Function2/8(psi_dot)
  Rate Transition2/1 -> Difference13/1, Add4/2
  Rate Transition3/1 -> Add4/1
  Rate Transition4/1 -> MATLAB Function2/6(phi_dot), Add5/1
  Data Type Conversion/1 -> Rate Transition4/1
  Data Type Conversion1/1 -> Rate Transition3/1
  Data Type Conversion2/1 -> Rate Transition/1
  Data Type Conversion3/1 -> Rate Transition1/1
  Gain/1 -> Display6/1  "u2chen10"
  Constant1/1 -> MATLAB Function2/15(K1)
  Constant2/1 -> MATLAB Function2/16(K2)
  Constant3/1 -> MATLAB Function2/10(alpha)
  Constant4/1 -> MATLAB Function2/11(beta)
  Constant5/1 -> MATLAB Function2/12(gamma)
  Constant6/1 -> MATLAB Function2/13(mu)
  Constant7/1 -> MATLAB Function2/14(r)
  Constant8/1 -> MATLAB Function2/9(s_integ_max)

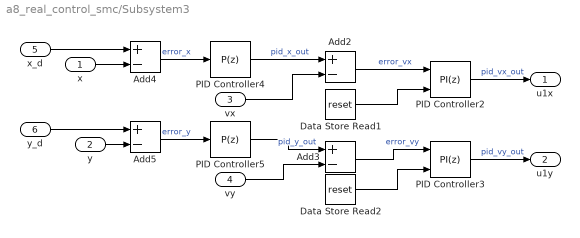
== system a8_real_control_smc/Subsystem3 ==
  x : Inport
  y : Inport  Port=2
  vx : Inport  Port=3
  vy : Inport  Port=4
  x_d : Inport  Port=5
  y_d : Inport  Port=6
  Add{2..5} (4 alike) : Sum  Inputs=+-
  Data Store Read1 : DataStoreRead  DataStoreName=reset  IndexOptions=Index vector (dialog)  Indices=1  OutputSizes=1
  Data Store Read2 : DataStoreRead  DataStoreName=reset  IndexOptions=Index vector (dialog)  Indices=1  OutputSizes=1
  PID Controller2 : slpidlib/PID Controller  Controller=PI  Form=Parallel  TimeDomain=Discrete-time  UseExternalTs=off  SampleTime=-1  IntegratorMethod=Forward Euler  FilterMethod=Forward Euler  ControllerParametersSource=internal  P=0.1  I=0.01  UseKiTs=off  D=0.947452162670561  N=36.1071689779307  UseFilter=on  TunerSelectOption=Transfer Function Based (PID Tuner App)  InitialConditionSource=internal  InitialConditionForIntegrator=0  InitialConditionForFilter=0  DifferentiatorICPrevScaledInput=0  ExternalReset=level  TrackingMode=off  Kt=1  LimitOutput=on  SatLimitsSource=internal  UpperSaturationLimit=1  LowerSaturationLimit=-1  LinearizeAsGain=off  AntiWindupMode=none  Kb=1  LimitIntegrator=off  UpperIntegratorSaturationLimit=inf  LowerIntegratorSaturationLimit=-inf  POutMin=[]  POutMax=[]  IOutMin=[]  IOutMax=[]  DOutMin=[]  DOutMax=[]  NOutMin=[]  NOutMax=[]  SumOutMin=[]  SumOutMax=[]  SaturationOutMin=[]  SaturationOutMax=[]  PParamMin=[]  PParamMax=[]  IParamMin=[]  IParamMax=[]  DParamMin=[]  DParamMax=[]  NParamMin=[]  NParamMax=[]  KbParamMin=[]  KbParamMax=[]  KtParamMin=[]  KtParamMax=[]  KbOutMin=[]  KbOutMax=[]  KtOutMin=[]  KtOutMax=[]  IntegratorOutMin=[]  IntegratorOutMax=[]  FilterOutMin=[]  FilterOutMax=[]  SumI1OutMin=[]  SumI1OutMax=[]  SumI2OutMin=[]  SumI2OutMax=[]  SumI3OutMin=[]  SumI3OutMax=[]  SumI4OutMin=[]  SumI4OutMax=[]  SumDOutMin=[]  SumDOutMax=[]  DifferentiatorOutMin=[]  DifferentiatorOutMax=[]  FilterDiffOutCoefMin=[]  FilterDiffOutCoefMax=[]  ReciprocalOutMin=[]  ReciprocalOutMax=[]  SumDenOutMin=[]  SumDenOutMax=[]  SumNumOutMin=[]  SumNumOutMax=[]  DivideOutMin=[]  DivideOutMax=[]  UdiffTsProdOutMin=[]  UdiffTsProdOutMax=[]  NTsProdOutMin=[]  NTsProdOutMax=[]  UintegralTsProdOutMin=[]  UintegralTsProdOutMax=[]  UngainTsProdOutMin=[]  UngainTsProdOutMax=[]  ClampingZeroOutDataTypeStr=Inherit: Inherit via back propagation  ClampingZeroOutMin=[]  ClampingZeroOutMax=[]  FilterDenConstantOutDataTypeStr=Inherit: Inherit via back propagation  FilterDenConstantOutMin=[]  FilterDenConstantOutMax=[]  PCopyOutDataTypeStr=Inherit: Inherit via back propagation  PCopyOutMin=[]  PCopyOutMax=[]  NCopyOutDataTypeStr=Inherit: Inherit via back propagation  NCopyOutMin=[]  NCopyOutMax=[]  IntegratorContinuousStateAttributes=''  IntegratorStateMustResolveToSignalObject=off  IntegratorRTWStateStorageClass=Auto  FilterContinuousStateAttributes=''  FilterStateMustResolveToSignalObject=off  FilterRTWStateStorageClass=Auto  ParallelPVariant=InternalParameters  IdealPVariant=Disabled  IVariant=InternalParameters  DVariant=Disabled  IntegratorVariant=Discrete  SatVariant=Enabled  AWVariant=Passthrough  PCopyVariant=Disabled  TRVariant=Disabled  FdbkBlocksVariant=Forward  IdealPFdbkVariant=Disabled  SatFdbkVariant=Disabled  DerivativeFilterVariant=Disabled  NVariant=Disabled  NCopyVariant=Disabled_SignalSpec  FilterICVariant=Disabled  IntegratorICVariant=InternalICs  ExternalResetVariant=ExternalReset  TRSumVariant=Passthrough  SumFdbkVariant=Disabled  SumVariant=Sum_PI  TsampFilterVariant=InternalTs  TsampNgainVariant=Passthrough  TsampIntegralVariant=Disabled_SignalSpec  ExternalSaturationOutDataTypeStr=Inherit: Same as second input
  PID Controller3 : slpidlib/PID Controller  Controller=PI  Form=Parallel  TimeDomain=Discrete-time  UseExternalTs=off  SampleTime=-1  IntegratorMethod=Forward Euler  FilterMethod=Forward Euler  ControllerParametersSource=internal  P=0.1  I=0.01  UseKiTs=off  D=0  N=10  UseFilter=off  TunerSelectOption=Transfer Function Based (PID Tuner App)  InitialConditionSource=internal  InitialConditionForIntegrator=0  InitialConditionForFilter=0  DifferentiatorICPrevScaledInput=0  ExternalReset=level  TrackingMode=off  Kt=1  LimitOutput=on  SatLimitsSource=internal  UpperSaturationLimit=1  LowerSaturationLimit=-1  LinearizeAsGain=off  AntiWindupMode=none  Kb=1  LimitIntegrator=off  UpperIntegratorSaturationLimit=inf  LowerIntegratorSaturationLimit=-inf  POutMin=[]  POutMax=[]  IOutMin=[]  IOutMax=[]  DOutMin=[]  DOutMax=[]  NOutMin=[]  NOutMax=[]  SumOutMin=[]  SumOutMax=[]  SaturationOutMin=[]  SaturationOutMax=[]  PParamMin=[]  PParamMax=[]  IParamMin=[]  IParamMax=[]  DParamMin=[]  DParamMax=[]  NParamMin=[]  NParamMax=[]  KbParamMin=[]  KbParamMax=[]  KtParamMin=[]  KtParamMax=[]  KbOutMin=[]  KbOutMax=[]  KtOutMin=[]  KtOutMax=[]  IntegratorOutMin=[]  IntegratorOutMax=[]  FilterOutMin=[]  FilterOutMax=[]  SumI1OutMin=[]  SumI1OutMax=[]  SumI2OutMin=[]  SumI2OutMax=[]  SumI3OutMin=[]  SumI3OutMax=[]  SumI4OutMin=[]  SumI4OutMax=[]  SumDOutMin=[]  SumDOutMax=[]  DifferentiatorOutMin=[]  DifferentiatorOutMax=[]  FilterDiffOutCoefMin=[]  FilterDiffOutCoefMax=[]  ReciprocalOutMin=[]  ReciprocalOutMax=[]  SumDenOutMin=[]  SumDenOutMax=[]  SumNumOutMin=[]  SumNumOutMax=[]  DivideOutMin=[]  DivideOutMax=[]  UdiffTsProdOutMin=[]  UdiffTsProdOutMax=[]  NTsProdOutMin=[]  NTsProdOutMax=[]  UintegralTsProdOutMin=[]  UintegralTsProdOutMax=[]  UngainTsProdOutMin=[]  UngainTsProdOutMax=[]  ClampingZeroOutDataTypeStr=Inherit: Inherit via back propagation  ClampingZeroOutMin=[]  ClampingZeroOutMax=[]  FilterDenConstantOutDataTypeStr=Inherit: Inherit via back propagation  FilterDenConstantOutMin=[]  FilterDenConstantOutMax=[]  PCopyOutDataTypeStr=Inherit: Inherit via back propagation  PCopyOutMin=[]  PCopyOutMax=[]  NCopyOutDataTypeStr=Inherit: Inherit via back propagation  NCopyOutMin=[]  NCopyOutMax=[]  IntegratorContinuousStateAttributes=''  IntegratorStateMustResolveToSignalObject=off  IntegratorRTWStateStorageClass=Auto  FilterContinuousStateAttributes=''  FilterStateMustResolveToSignalObject=off  FilterRTWStateStorageClass=Auto  ParallelPVariant=InternalParameters  IdealPVariant=Disabled  IVariant=InternalParameters  DVariant=Disabled  IntegratorVariant=Discrete  SatVariant=Enabled  AWVariant=Passthrough  PCopyVariant=Disabled  TRVariant=Disabled  FdbkBlocksVariant=Forward  IdealPFdbkVariant=Disabled  SatFdbkVariant=Disabled  DerivativeFilterVariant=Disabled  NVariant=Disabled  NCopyVariant=Disabled_SignalSpec  FilterICVariant=Disabled  IntegratorICVariant=InternalICs  ExternalResetVariant=ExternalReset  TRSumVariant=Passthrough  SumFdbkVariant=Disabled  SumVariant=Sum_PI  TsampFilterVariant=InternalTs  TsampNgainVariant=Passthrough  TsampIntegralVariant=Disabled_SignalSpec  ExternalSaturationOutDataTypeStr=Inherit: Same as second input
  PID Controller4 : slpidlib/PID Controller  Controller=P  Form=Parallel  TimeDomain=Discrete-time  UseExternalTs=off  SampleTime=-1  IntegratorMethod=Forward Euler  FilterMethod=Forward Euler  ControllerParametersSource=internal  P=0.8  I=0.02  UseKiTs=off  D=0.245723815521348  N=312.971612169429  UseFilter=on  TunerSelectOption=Transfer Function Based (PID Tuner App)  InitialConditionSource=internal  InitialConditionForIntegrator=0  InitialConditionForFilter=0  DifferentiatorICPrevScaledInput=0  ExternalReset=none  TrackingMode=off  Kt=1  LimitOutput=on  SatLimitsSource=internal  UpperSaturationLimit=10  LowerSaturationLimit=-10  LinearizeAsGain=off  AntiWindupMode=none  Kb=1  LimitIntegrator=off  UpperIntegratorSaturationLimit=inf  LowerIntegratorSaturationLimit=-inf  POutMin=[]  POutMax=[]  IOutMin=[]  IOutMax=[]  DOutMin=[]  DOutMax=[]  NOutMin=[]  NOutMax=[]  SumOutMin=[]  SumOutMax=[]  SaturationOutMin=[]  SaturationOutMax=[]  PParamMin=[]  PParamMax=[]  IParamMin=[]  IParamMax=[]  DParamMin=[]  DParamMax=[]  NParamMin=[]  NParamMax=[]  KbParamMin=[]  KbParamMax=[]  KtParamMin=[]  KtParamMax=[]  KbOutMin=[]  KbOutMax=[]  KtOutMin=[]  KtOutMax=[]  IntegratorOutMin=[]  IntegratorOutMax=[]  FilterOutMin=[]  FilterOutMax=[]  SumI1OutMin=[]  SumI1OutMax=[]  SumI2OutMin=[]  SumI2OutMax=[]  SumI3OutMin=[]  SumI3OutMax=[]  SumI4OutMin=[]  SumI4OutMax=[]  SumDOutMin=[]  SumDOutMax=[]  DifferentiatorOutMin=[]  DifferentiatorOutMax=[]  FilterDiffOutCoefMin=[]  FilterDiffOutCoefMax=[]  ReciprocalOutMin=[]  ReciprocalOutMax=[]  SumDenOutMin=[]  SumDenOutMax=[]  SumNumOutMin=[]  SumNumOutMax=[]  DivideOutMin=[]  DivideOutMax=[]  UdiffTsProdOutMin=[]  UdiffTsProdOutMax=[]  NTsProdOutMin=[]  NTsProdOutMax=[]  UintegralTsProdOutMin=[]  UintegralTsProdOutMax=[]  UngainTsProdOutMin=[]  UngainTsProdOutMax=[]  ClampingZeroOutDataTypeStr=Inherit: Inherit via back propagation  ClampingZeroOutMin=[]  ClampingZeroOutMax=[]  FilterDenConstantOutDataTypeStr=Inherit: Inherit via back propagation  FilterDenConstantOutMin=[]  FilterDenConstantOutMax=[]  PCopyOutDataTypeStr=Inherit: Inherit via back propagation  PCopyOutMin=[]  PCopyOutMax=[]  NCopyOutDataTypeStr=Inherit: Inherit via back propagation  NCopyOutMin=[]  NCopyOutMax=[]  IntegratorContinuousStateAttributes=''  IntegratorStateMustResolveToSignalObject=off  IntegratorRTWStateStorageClass=Auto  FilterContinuousStateAttributes=''  FilterStateMustResolveToSignalObject=off  FilterRTWStateStorageClass=Auto  ParallelPVariant=InternalParameters  IdealPVariant=Disabled  IVariant=Disabled  DVariant=Disabled  IntegratorVariant=Disabled  SatVariant=Enabled  AWVariant=Disabled  PCopyVariant=Disabled  TRVariant=Disabled  FdbkBlocksVariant=Forward  IdealPFdbkVariant=Disabled  SatFdbkVariant=Disabled  DerivativeFilterVariant=Disabled  NVariant=Disabled  NCopyVariant=Disabled_SignalSpec  FilterICVariant=Disabled  IntegratorICVariant=Disabled  ExternalResetVariant=Disabled  TRSumVariant=Passthrough  SumFdbkVariant=Disabled  SumVariant=Passthrough_P  TsampFilterVariant=InternalTs  TsampNgainVariant=Passthrough  TsampIntegralVariant=Disabled_SignalSpec  ExternalSaturationOutDataTypeStr=Inherit: Same as second input
  PID Controller5 : slpidlib/PID Controller  Controller=P  Form=Parallel  TimeDomain=Discrete-time  UseExternalTs=off  SampleTime=-1  IntegratorMethod=Forward Euler  FilterMethod=Forward Euler  ControllerParametersSource=internal  P=0.8  I=pid_y_i  UseKiTs=off  D=0.377572647695254  N=483.906486380362  UseFilter=on  TunerSelectOption=Transfer Function Based (PID Tuner App)  InitialConditionSource=internal  InitialConditionForIntegrator=0  InitialConditionForFilter=0  DifferentiatorICPrevScaledInput=0  ExternalReset=none  TrackingMode=off  Kt=1  LimitOutput=on  SatLimitsSource=internal  UpperSaturationLimit=10  LowerSaturationLimit=-10  LinearizeAsGain=off  AntiWindupMode=none  Kb=1  LimitIntegrator=off  UpperIntegratorSaturationLimit=inf  LowerIntegratorSaturationLimit=-inf  POutMin=[]  POutMax=[]  IOutMin=[]  IOutMax=[]  DOutMin=[]  DOutMax=[]  NOutMin=[]  NOutMax=[]  SumOutMin=[]  SumOutMax=[]  SaturationOutMin=[]  SaturationOutMax=[]  PParamMin=[]  PParamMax=[]  IParamMin=[]  IParamMax=[]  DParamMin=[]  DParamMax=[]  NParamMin=[]  NParamMax=[]  KbParamMin=[]  KbParamMax=[]  KtParamMin=[]  KtParamMax=[]  KbOutMin=[]  KbOutMax=[]  KtOutMin=[]  KtOutMax=[]  IntegratorOutMin=[]  IntegratorOutMax=[]  FilterOutMin=[]  FilterOutMax=[]  SumI1OutMin=[]  SumI1OutMax=[]  SumI2OutMin=[]  SumI2OutMax=[]  SumI3OutMin=[]  SumI3OutMax=[]  SumI4OutMin=[]  SumI4OutMax=[]  SumDOutMin=[]  SumDOutMax=[]  DifferentiatorOutMin=[]  DifferentiatorOutMax=[]  FilterDiffOutCoefMin=[]  FilterDiffOutCoefMax=[]  ReciprocalOutMin=[]  ReciprocalOutMax=[]  SumDenOutMin=[]  SumDenOutMax=[]  SumNumOutMin=[]  SumNumOutMax=[]  DivideOutMin=[]  DivideOutMax=[]  UdiffTsProdOutMin=[]  UdiffTsProdOutMax=[]  NTsProdOutMin=[]  NTsProdOutMax=[]  UintegralTsProdOutMin=[]  UintegralTsProdOutMax=[]  UngainTsProdOutMin=[]  UngainTsProdOutMax=[]  ClampingZeroOutDataTypeStr=Inherit: Inherit via back propagation  ClampingZeroOutMin=[]  ClampingZeroOutMax=[]  FilterDenConstantOutDataTypeStr=Inherit: Inherit via back propagation  FilterDenConstantOutMin=[]  FilterDenConstantOutMax=[]  PCopyOutDataTypeStr=Inherit: Inherit via back propagation  PCopyOutMin=[]  PCopyOutMax=[]  NCopyOutDataTypeStr=Inherit: Inherit via back propagation  NCopyOutMin=[]  NCopyOutMax=[]  IntegratorContinuousStateAttributes=''  IntegratorStateMustResolveToSignalObject=off  IntegratorRTWStateStorageClass=Auto  FilterContinuousStateAttributes=''  FilterStateMustResolveToSignalObject=off  FilterRTWStateStorageClass=Auto  ParallelPVariant=InternalParameters  IdealPVariant=Disabled  IVariant=Disabled  DVariant=Disabled  IntegratorVariant=Disabled  SatVariant=Enabled  AWVariant=Disabled  PCopyVariant=Disabled  TRVariant=Disabled  FdbkBlocksVariant=Forward  IdealPFdbkVariant=Disabled  SatFdbkVariant=Disabled  DerivativeFilterVariant=Disabled  NVariant=Disabled  NCopyVariant=Disabled_SignalSpec  FilterICVariant=Disabled  IntegratorICVariant=Disabled  ExternalResetVariant=Disabled  TRSumVariant=Passthrough  SumFdbkVariant=Disabled  SumVariant=Passthrough_P  TsampFilterVariant=InternalTs  TsampNgainVariant=Passthrough  TsampIntegralVariant=Disabled_SignalSpec  ExternalSaturationOutDataTypeStr=Inherit: Same as second input
  u1x : Outport
  u1y : Outport  Port=2
  wires:
  PID Controller5/1 -> Add3/1  "pid_y_out"
  Data Store Read2/1 -> PID Controller3/2
  x_d/1 -> Add4/1
  PID Controller3/1 -> u1y/1  "pid_vy_out"
  Add4/1 -> PID Controller4/1  "error_x"
  vy/1 -> Add3/2
  vx/1 -> Add2/2
  PID Controller4/1 -> Add2/1  "pid_x_out"
  Add3/1 -> PID Controller3/1  "error_vy"
  PID Controller2/1 -> u1x/1  "pid_vx_out"
  Add2/1 -> PID Controller2/1  "error_vx"
  Add5/1 -> PID Controller5/1  "error_y"
  y_d/1 -> Add5/1
  Data Store Read1/1 -> PID Controller2/2
  x/1 -> Add4/2
  y/1 -> Add5/2

== system a8_real_control_smc/F2pwm/F2pwmFcn ==
  F : Inport
  ThrustFactor : Inport  Port=2
  Fcn : Fcn  Expr=(sqrt((u(1)+((1-u(2))^2)/(4*u(2)))/u(2))-(1-u(2))/(2*u(2)))
  Mux : Mux  Inputs=2
  pwm : Outport  OutDataTypeStr=double  VectorParamsAs1DForOutWhenUnconnected=off
  wires:
  Fcn/1 -> pwm/1
  Mux/1 -> Fcn/1
  F/1 -> Mux/1
  ThrustFactor/1 -> Mux/2

== system a8_real_control_smc/F2pwm1/F2pwmFcn ==
  F : Inport
  ThrustFactor : Inport  Port=2
  Fcn : Fcn  Expr=(sqrt((u(1)+((1-u(2))^2)/(4*u(2)))/u(2))-(1-u(2))/(2*u(2)))
  Mux : Mux  Inputs=2
  pwm : Outport  OutDataTypeStr=double  VectorParamsAs1DForOutWhenUnconnected=off
  wires:
  ThrustFactor/1 -> Mux/2
  F/1 -> Mux/1
  Mux/1 -> Fcn/1
  Fcn/1 -> pwm/1

== system a8_real_control_smc/F2pwm2/F2pwmFcn ==
  F : Inport
  ThrustFactor : Inport  Port=2
  Fcn : Fcn  Expr=(sqrt((u(1)+((1-u(2))^2)/(4*u(2)))/u(2))-(1-u(2))/(2*u(2)))
  Mux : Mux  Inputs=2
  pwm : Outport  OutDataTypeStr=double  VectorParamsAs1DForOutWhenUnconnected=off
  wires:
  Fcn/1 -> pwm/1
  Mux/1 -> Fcn/1
  F/1 -> Mux/1
  ThrustFactor/1 -> Mux/2

== system a8_real_control_smc/F2pwm3/F2pwmFcn ==
  F : Inport
  ThrustFactor : Inport  Port=2
  Fcn : Fcn  Expr=(sqrt((u(1)+((1-u(2))^2)/(4*u(2)))/u(2))-(1-u(2))/(2*u(2)))
  Mux : Mux  Inputs=2
  pwm : Outport  OutDataTypeStr=double  VectorParamsAs1DForOutWhenUnconnected=off
  wires:
  ThrustFactor/1 -> Mux/2
  F/1 -> Mux/1
  Mux/1 -> Fcn/1
  Fcn/1 -> pwm/1

== system a8_real_control_smc/FlightMode_z/Subsystem 1 ==
  Inport2 : Inport
  Action Port : ActionPort  ActionPortLabel=case [ 0 ]:
  Out1 : Outport  VectorParamsAs1DForOutWhenUnconnected=off
  wires:
  Inport2/1 -> Out1/1

== system a8_real_control_smc/FlightMode_z/Subsystem 2 ==
  In1 : Inport
  Action Port : ActionPort  ActionPortLabel=case [ 1 ]:
  Out1 : Outport  VectorParamsAs1DForOutWhenUnconnected=off
  wires:
  In1/1 -> Out1/1

== system a8_real_control_smc/FlightMode_z/Subsystem 3 ==
  In1 : Inport
  Action Port : ActionPort  ActionPortLabel=default:
  Out1 : Outport  VectorParamsAs1DForOutWhenUnconnected=off
  wires:
  In1/1 -> Out1/1

== system a8_real_control_smc/RC_cmd/ArmingControl1 ==
  ch7 : Inport
  Compare To Constant1 : simulink/Logic and Bit Operations/Compare To Constant  relop=<=  const=uint16(1200)  OutDataTypeStr=boolean
  ARM Control : Outport  OutDataTypeStr=boolean  VectorParamsAs1DForOutWhenUnconnected=off
  wires:
  Compare To Constant1/1 -> ARM Control/1
  ch7/1 -> Compare To Constant1/1

== system a8_real_control_smc/RC_cmd/ArmingControl2 ==
  ch6 : Inport
  Compare To Constant1 : simulink/Logic and Bit Operations/Compare To Constant  relop=>=  const=uint16(1800)  OutDataTypeStr=boolean
  ARM Control : Outport  OutDataTypeStr=boolean  VectorParamsAs1DForOutWhenUnconnected=off
  wires:
  ch6/1 -> Compare To Constant1/1
  Compare To Constant1/1 -> ARM Control/1

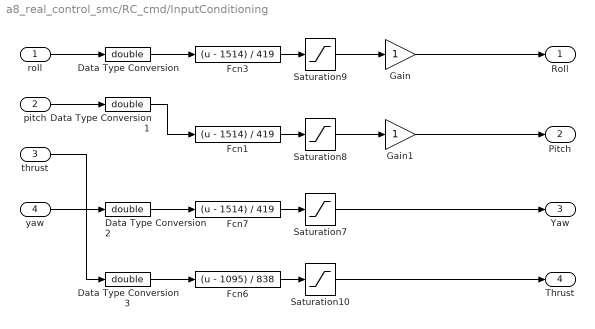
== system a8_real_control_smc/RC_cmd/InputConditioning ==
  roll : Inport
  pitch : Inport  Port=2
  thrust : Inport  Port=3
  yaw : Inport  Port=4
  Data Type Conversion{,1..3} (4 alike) : DataTypeConversion  OutDataTypeStr=double  SaturateOnIntegerOverflow=off  RndMeth=Floor
  Fcn1 : Fcn  Expr=(u - 1514) / 419
  Fcn3 : Fcn  Expr=(u - 1514) / 419
  Fcn6 : Fcn  Expr=(u - 1095) / 838
  Fcn7 : Fcn  Expr=(u - 1514) / 419
  Gain : Gain
  Gain1 : Gain
  Saturation10 : Saturate  UpperLimit=1  LowerLimit=0
  Saturation7 : Saturate  UpperLimit=1  LowerLimit=-1
  Saturation8 : Saturate  UpperLimit=1  LowerLimit=-1
  Saturation9 : Saturate  UpperLimit=1  LowerLimit=-1
  Roll : Outport  VectorParamsAs1DForOutWhenUnconnected=off
  Pitch : Outport  Port=2  VectorParamsAs1DForOutWhenUnconnected=off
  Yaw : Outport  Port=3  VectorParamsAs1DForOutWhenUnconnected=off
  Thrust : Outport  Port=4  VectorParamsAs1DForOutWhenUnconnected=off
  wires:
  Data Type Conversion3/1 -> Fcn6/1
  Data Type Conversion2/1 -> Fcn7/1
  Data Type Conversion1/1 -> Fcn1/1
  Data Type Conversion/1 -> Fcn3/1
  roll/1 -> Data Type Conversion/1
  pitch/1 -> Data Type Conversion1/1
  yaw/1 -> Data Type Conversion2/1
  Fcn7/1 -> Saturation7/1
  Saturation9/1 -> Gain/1
  Fcn1/1 -> Saturation8/1
  Fcn3/1 -> Saturation9/1
  thrust/1 -> Data Type Conversion3/1
  Fcn6/1 -> Saturation10/1
  Saturation8/1 -> Gain1/1
  Saturation7/1 -> Yaw/1
  Saturation10/1 -> Thrust/1
  Gain/1 -> Roll/1
  Gain1/1 -> Pitch/1

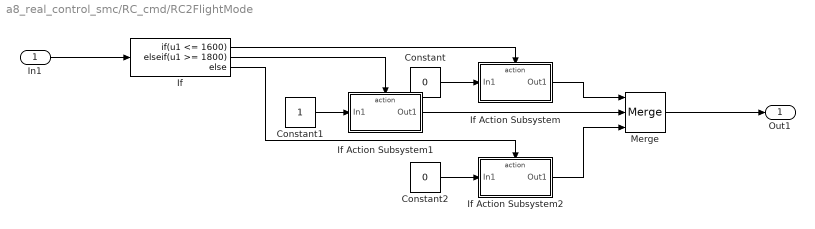
== system a8_real_control_smc/RC_cmd/RC2FlightMode ==
  In1 : Inport
  Constant : Constant  Value=0  OutDataTypeStr=uint8
  Constant1 : Constant  OutDataTypeStr=uint8
  Constant2 : Constant  Value=0  OutDataTypeStr=uint8
  If : If  IfExpression=u1 <= 1600  ElseIfExpressions=u1 >= 1800
  If Action Subsystem : Subsystem  TreatAsAtomicUnit=on
  If Action Subsystem1 : Subsystem  TreatAsAtomicUnit=on
  If Action Subsystem2 : Subsystem  TreatAsAtomicUnit=on
  Merge : Merge  Inputs=3  InitialOutput=[0]
  Out1 : Outport
  wires:
  If Action Subsystem2/1(Out1) -> Merge/3
  If/3 -> If Action Subsystem2/Action
  If Action Subsystem1/1(Out1) -> Merge/2
  Constant/1 -> If Action Subsystem/1(In1)
  If/2 -> If Action Subsystem1/Action
  Constant1/1 -> If Action Subsystem1/1(In1)
  If Action Subsystem/1(Out1) -> Merge/1
  If/1 -> If Action Subsystem/Action
  Merge/1 -> Out1/1
  Constant2/1 -> If Action Subsystem2/1(In1)
  In1/1 -> If/1

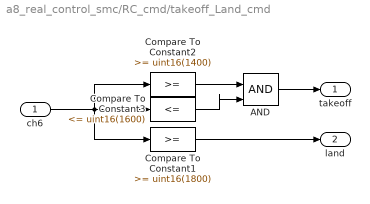
== system a8_real_control_smc/RC_cmd/takeoff_Land_cmd ==
  ch6 : Inport
  AND : Logic  IconShape=distinctive  AllPortsSameDT=off  OutDataTypeStr=boolean
  Compare To Constant1 : simulink/Logic and Bit Operations/Compare To Constant  relop=>=  const=uint16(1800)  OutDataTypeStr=boolean
  Compare To Constant2 : simulink/Logic and Bit Operations/Compare To Constant  relop=>=  const=uint16(1400)  OutDataTypeStr=boolean
  Compare To Constant3 : simulink/Logic and Bit Operations/Compare To Constant  relop=<=  const=uint16(1600)  OutDataTypeStr=boolean
  takeoff : Outport  OutDataTypeStr=boolean  VectorParamsAs1DForOutWhenUnconnected=off
  land : Outport  Port=2  OutDataTypeStr=boolean  VectorParamsAs1DForOutWhenUnconnected=off
  wires:
  Compare To Constant1/1 -> land/1
  ch6/1 -> Compare To Constant1/1, Compare To Constant3/1, Compare To Constant2/1
  Compare To Constant2/1 -> AND/1
  Compare To Constant3/1 -> AND/2
  AND/1 -> takeoff/1

== system a8_real_control_smc/RC_cmd/RC2FlightMode/If Action Subsystem ==
  In1 : Inport
  Action Port : ActionPort  ActionPortLabel=if(u1 <= 1600)
  Out1 : Outport
  wires:
  In1/1 -> Out1/1

== system a8_real_control_smc/RC_cmd/RC2FlightMode/If Action Subsystem1 ==
  In1 : Inport
  Action Port : ActionPort  ActionPortLabel=elseif(u1 >= 1800)
  Out1 : Outport
  wires:
  In1/1 -> Out1/1
